simulink model "PIcontrol"  (R2018a)
settings: Solver=VariableStepAuto  StartTime=0.0  StopTime=2  RelTol=1e-3
libraries: powerlib x10, powerlib_meascontrol x1
settings Model: Creator=enes_  LastModifiedBy=enes_

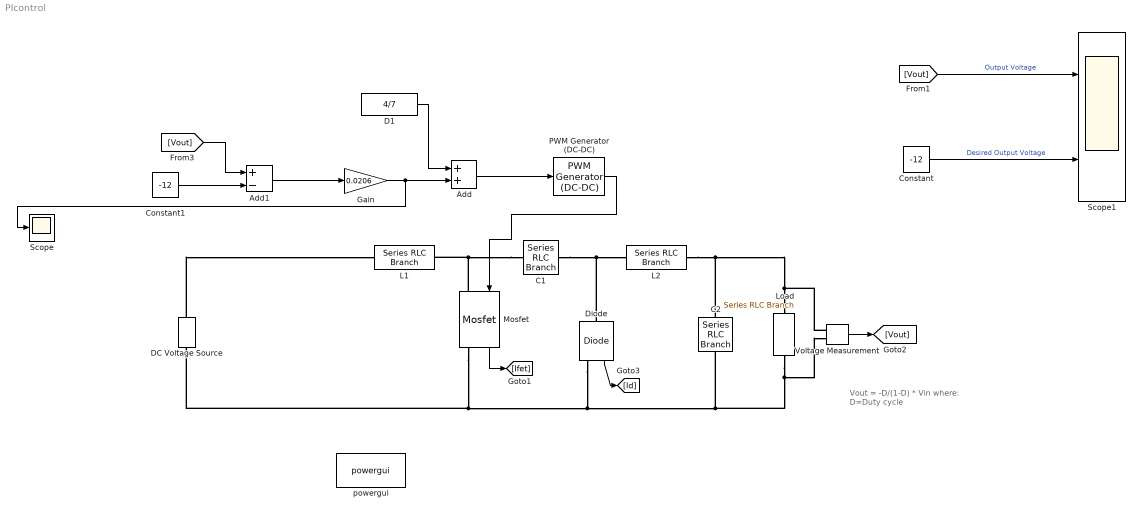
== system PIcontrol ==
  note: Vout = -D/(1-D) * Vin
      | where: D=Duty cycle
  Add : Sum
  Add1 : Sum  Inputs=+-
  C1 : powerlib/Elements/Series RLC Branch  LConnTagsString=__new0  RConnTagsString=__new0  BranchType=C  Resistance=1e-4  Inductance=200e-6  SetiL0=off  InitialCurrent=0  Capacitance=22e-6  Setx0=off  InitialVoltage=40  Measurements=None
  C2 : powerlib/Elements/Series RLC Branch  LConnTagsString=__new0  RConnTagsString=__new0  BranchType=C  Resistance=1e-4  Inductance=200e-6  SetiL0=off  InitialCurrent=0  Capacitance=47e-6  Setx0=on  InitialVoltage=-5  Measurements=None
  Constant : Constant  Value=-12
  Constant1 : Constant  Value=-12
  D1 : Constant  Value=4/7
  DC Voltage Source : powerlib/Electrical Sources/DC Voltage Source  Amplitude=9  Measurements=None
  Diode : powerlib/Power Electronics/Diode  Ron=1e-3  Lon=0  Vf=0  IC=0  UseSnubber=off  Rs=inf  Cs=inf  Measurements=on
  Gain : Gain  Gain=0.0206
  L1 : powerlib/Elements/Series RLC Branch  LConnTagsString=__new0  RConnTagsString=__new0  BranchType=L  Resistance=1e-3  Inductance=15e-6  SetiL0=on  InitialCurrent=4  Capacitance=1e-6  Setx0=off  InitialVoltage=0  Measurements=Branch current
  L2 : powerlib/Elements/Series RLC Branch  LConnTagsString=__new0  RConnTagsString=__new0  BranchType=L  Resistance=1e-3  Inductance=33e-6  SetiL0=on  InitialCurrent=-10  Capacitance=1e-6  Setx0=off  InitialVoltage=0  Measurements=Branch current
  Load : powerlib/Elements/Series RLC Branch  LConnTagsString=__new0  RConnTagsString=__new0  BranchType=R  Resistance=4  Inductance=200e-6  SetiL0=off  InitialCurrent=0  Capacitance=400e-6  Setx0=off  InitialVoltage=0  Measurements=None
  Mosfet : powerlib/Power Electronics/Mosfet  Ron=1e-3  Lon=0  Rd=1e-3  Vfd=0  IC=0  Rs=1e6  Cs=inf  Measurements=on
  PWM Generator (DC-DC) : powerlib_meascontrol/Pulse & Signal Generators/PWM Generator (DC-DC)  Fsw=100e3  Ts=0
  Scope : Scope
  Scope1 : Scope  NumInputPorts=2
  Voltage Measurement : powerlib/Measurements/Voltage Measurement  PhasorSimulation=off  OutputType=Complex  PSBequivalent=0
  powergui : powerlib/powergui  Priority=1  SimulationMode=Continuous  SampleTime=50e-6  frequency=60  Iterations=50  frequencyindice=0  Pbase=100e6  ErrMax=1e-4  UnitsV=kV  UnitsW=MW  buscounter=0  FunctionMessages=off  echomessages=off  EnableUseOfTLC=off  CurrentSourceSwitches=off  DisableSnubberDevices=off  DisableRonSwitches=off  DisableVfSwitches=off  DisplayEquations=off  SolverType=Tustin/Backward Euler (TBE)  Interpol=off  ExternalGateDelay=off  methode=off  Ts=100  x0status=blocks  SPID=off  SwTol=0  HookPort=off  RestoreLinks=warning  ResistiveCurrentMeasurement=off  Frange=[0:2:500]  Ylog=off  Xlog=on  ShowGrid=off  save=off  variable=ZData  structure=0  ZoomFFT=off  StartTime=0.0  cycles=1  DisplayStyle=1  fundamental=60  FreqAxis=off  MaxFrequency=1000  frequencyindicesteady=1  RmsSteady=1  display=off
  wires:
  Mosfet/1 -> [Ifet]
  PWM Generator (DC-DC)/1 -> Mosfet/1
  Diode/1 -> [Id]
  Voltage Measurement/1 -> [Vout]
  [Vout] -> Scope1/1  "Output Voltage"
  [Vout] -> Add1/1
  Add/1 -> PWM Generator (DC-DC)/1
  Constant/1 -> Scope1/2  "Desired Output Voltage"
  D1/1 -> Add/1
  Constant1/1 -> Add1/2
  Add1/1 -> Gain/1
  Gain/1 -> Scope/1, Add/2
  connections:
  C1/RConn1 -- Diode/LConn1 -- L2/LConn1
  L2/RConn1 -- Voltage Measurement/LConn1 -- Load/LConn1 -- C2/LConn1
  Voltage Measurement/LConn2 -- Load/RConn1 -- DC Voltage Source/LConn1 -- Mosfet/RConn1 -- Diode/RConn1 -- C2/RConn1
  C1/LConn1 -- Mosfet/LConn1 -- L1/RConn1
  DC Voltage Source/RConn1 -- L1/LConn1
